simulink model "exp_9_1"  (R2020a)
settings: Solver=VariableStepAuto  StartTime=0.0  StopTime=10  RelTol=1e-3
libraries: dspsrcs4 x2
settings Model: Creator=Jamil  LastModifiedBy=Jamil

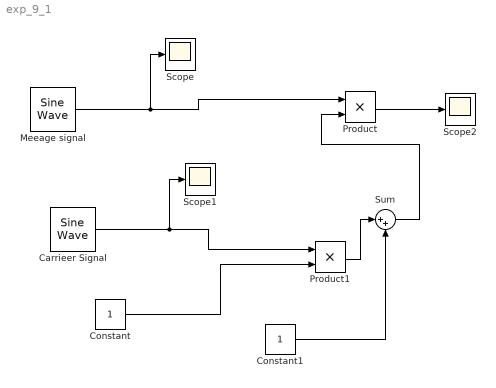
== system exp_9_1 ==
  Carrieer Signal : dspsrcs4/Sine Wave  Amplitude=5  Frequency=25  Phase=0  SampleMode=Discrete  OutComplex=Real  CompMethod=Trigonometric fcn  TableSize=Speed  SampleTime=1/5000  SamplesPerFrame=1  ResetState=Restart at time zero  OutputFrames=off  dataType=double  wordLen=16  udDataType=sfix(16)  fracBitsMode=Best precision  numFracBits=15  OutDataTypeStr=double  LastOutDataTypeStr=double
  Constant : Constant
  Constant1 : Constant
  Meeage signal : dspsrcs4/Sine Wave  Amplitude=5  Frequency=1  Phase=0  SampleMode=Discrete  OutComplex=Real  CompMethod=Trigonometric fcn  TableSize=Speed  SampleTime=1/5000  SamplesPerFrame=1  ResetState=Restart at time zero  OutputFrames=off  dataType=double  wordLen=16  udDataType=sfix(16)  fracBitsMode=Best precision  numFracBits=15  OutDataTypeStr=double  LastOutDataTypeStr=double
  Product : Product
  Product1 : Product
  Scope : Scope
  Scope1 : Scope
  Scope2 : Scope
  Sum : Sum  Inputs=|++
  wires:
  Carrieer Signal/1 -> Scope1/1, Product1/1
  Constant/1 -> Product1/2
  Constant1/1 -> Sum/2
  Product1/1 -> Sum/1
  Sum/1 -> Product/2
  Product/1 -> Scope2/1
  Meeage signal/1 -> Scope/1, Product/1
